simulink model "FourZones_STD2004_Buffalo_DenOcc"  (R2020a)
settings: Solver=FixedStepAuto  StartTime=20390400  StopTime=20563200  FixedStep=60  RelTol=1e-3
settings Model: Creator=zhelu  LastModifiedBy=yl3328

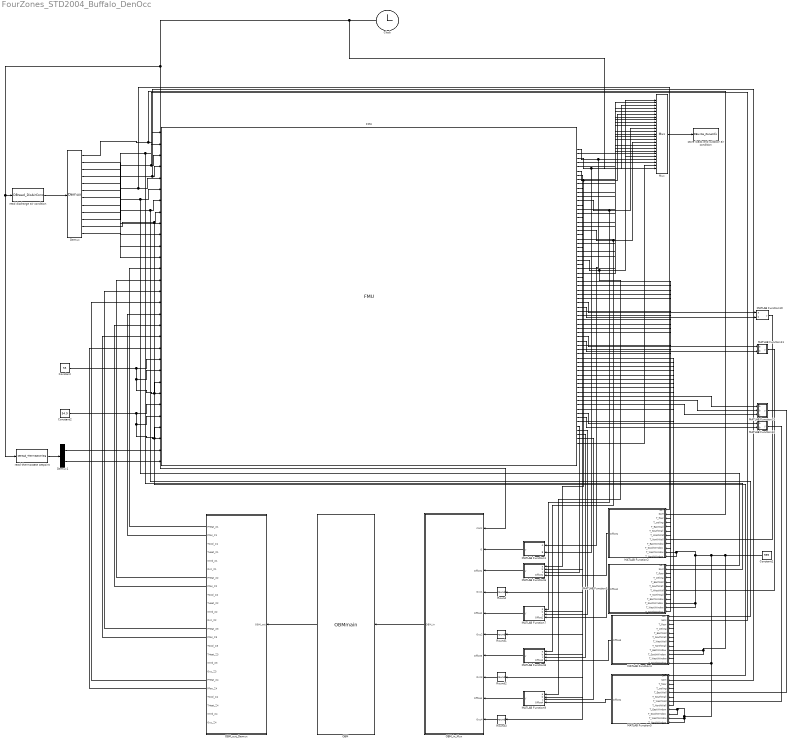
== system FourZones_STD2004_Buffalo_DenOcc ==
  Clock : Clock
  Constant : Constant  Value=55
  Constant1 : Constant  Value=999
  Constant2 : Constant  Value=54.9
  Demux : Demux  Outputs=12
  Demux1 : Demux  Outputs=2
  FMU : FMU  FMUName=ASHRAE901_OfficeMedium_STD2004_BuffaloBaseline_ARP_Cooling_dense.fmu  FMUMode=CoSimulation
      mask Type: ASHRAE901_OfficeMedium_STD2004_BuffaloBaseline.ARP_Cooling.idf [Co-Simulation, v2.0]
      mask Display:
      | disp('ASHRAE901_OfficeMedium_STD2004_BuffaloBaseline.ARP_Cooling.idf');
      | port_label('output',1,'T_out');
      | port_label('output',2,'DewpointT_out');
      | port_label('output',3,'RH_out');
      | port_label('output',4,'ConfRoom_Mid_2 ZN_SenLoads');
      | port_label('output',5,'ConfRoom_Mid_2 ZN_LatLoads');
      | port_label('output',6,'ConfRoom_Mid_2 ZN_Temp');
      | port_label('output',7,'ConfRoom_Mid_2 ZN_RadTemp');
      | port_label('output',8,'ConfRoom_Mid_2 ZN_DewpointT');
      | port_label('output',9,'ConfRoom_Mid_2 ZN_HumdRat');
      | port_label('output',10,'ConfRoom_Mid_2 ZN_Occ');
      | port_label('output',11,'EnclosedOffice_Mid_2 ZN_SenLoads');
      | port_label('output',12,'EnclosedOffice_Mid_2 ZN_LatLoads');
      | port_label('output',13,'EnclosedOffice_Mid_2 ZN_Temp');
      | port_label('output',14,'EnclosedOffice_Mid_2 ZN_RadTemp');
      | port_label('output',15,'EnclosedOffice_Mid_2 ZN_DewpointT');
      | port_label('output',16,'EnclosedOffice_Mid_2 ZN_HumdRat');
      | port_label('output',17,'EnclosedOffice_Mid_2 ZN_Occ');
      | port_label('output',18,'EnclosedOffice_Mid_5 ZN_SenLoads');
      | port_label('output',19,'EnclosedOffice_Mid_5 ZN_LatLoads');
      | port_label('output',20,'EnclosedOffice_Mid_5 ZN_Temp');
      | port_label('output',21,'EnclosedOffice_Mid_5 ZN_RadTemp');
      | port_label('output',22,'EnclosedOffice_Mid_5 ZN _DewpointT');
      | port_label('output',23,'EnclosedOffice_Mid_5 ZN_HumdRat');
      | port_label('output',24,'EnclosedOffice_Mid_5 ZN_Occ');
      | port_label('output',25,'OpenOffice_Mid_1 ZN_SenLoads');
      | port_label('output',26,'OpenOffice_Mid_1 ZN_LatLoads');
      | port_label('output',27,'OpenOffice_Mid_1 ZN_Temp');
      | port_label('output',28,'OpenOffice_Mid_1 ZN_RadTemp');
      | port_label('output',29,'OpenOffice_Mid_1 ZN_DewpointT');
      | port_label('output',30,'OpenOffice_Mid_1 ZN_HumdRat');
      | port_label('output',31,'OpenOffice_Mid_1 ZN_Occ');
      | port_label('output',32,'CONFROOM_MID_2_ZN_FLOOR_T');
      | port_label('output',33,'CONFROOM_MID_2_ZN_CEILING_T');
      | port_label('output',34,'CONFROOM_MID_2_ZN_WALL_EAST_T');
      | port_label('output',35,'CONFROOM_MID_2_ZN_WALL_SOUTH_T');
      | port_label('output',36,'CONFROOM_MID_2_ZN_WALL_WEST_T');
      | port_label('output',37,'CONFROOM_MID_2_ZN_WALL_NORTH_1_T');
      | port_label('output',38,'CONFROOM_MID_2_ZN_WALL_NORTH_2_T');
      | port_label('output',39,'CONFROOM_MID_2_ZN_WALL_EAST_WINDOW_T');
      | port_label('output',40,'CONFROOM_MID_2_ZN_WALL_SOUTH_WINDOW_T');
      | port_label('output',41,'ENCLOSEDOFFICE_MID_2_ZN_FLOOR_T');
      | port_label('output',42,'ENCLOSEDOFFICE_MID_2_ZN_CEILING_T');
      | port_label('output',43,'ENCLOSEDOFFICE_MID_2_ZN_WALL_EAST_T');
      | port_label('output',44,'ENCLOSEDOFFICE_MID_2_ZN_WALL_SOUTH_T');
      | port_label('output',45,'ENCLOSEDOFFICE_MID_2_ZN_WALL_WEST_1_T');
      | port_label('output',46,'ENCLOSEDOFFICE_MID_2_ZN_WALL_WEST_2_T');
      | port_label('output',47,'ENCLOSEDOFFICE_MID_2_ZN_WALL_NORTH_T');
      | port_label('output',48,'ENCLOSEDOFFICE_MID_2_ZN_WALL_NORTH_WINDOW_T');
      | port_label('output',49,'ENCLOSEDOFFICE_MID_2_ZN_WALL_EAST_WINDOW_T');
      | port_label('output',50,'ENCLOSEDOFFICE_MID_5_ZN_FLOOR_T');
      | port_label('output',51,'ENCLOSEDOFFICE_MID_5_ZN_CEILING_T');
      | port_label('output',52,'ENCLOSEDOFFICE_MID_5_ZN_WALL_EAST_T');
      | port_label('output',53,'ENCLOSEDOFFICE_MID_5_ZN_WALL_SOUTH_T');
      | port_label('output',54,'ENCLOSEDOFFICE_MID_5_ZN_WALL_WEST_T');
      | port_label('output',55,'ENCLOSEDOFFICE_MID_5_ZN_WALL_NORTH_T');
      | port_label('output',56,'ENCLOSEDOFFICE_MID_5_ZN_WALL_WEST_WINDOW_T');
      | port_label('output',57,'OPENOFFICE_MID_1_ZN_FLOOR_T');
      | port_label('output',58,'OPENOFFICE_MID_1_ZN_CEILING_T');
      | port_label('output',59,'OPENOFFICE_MID_1_ZN_WALL_EAST_1_T');
      | port_label('output',60,'OPENOFFICE_MID_1_ZN_WALL_EAST_2_T');
      | port_label('output',61,'OPENOFFICE_MID_1_ZN_WALL_EAST_3_T');
      | port_label('output',62,'OPENOFFICE_MID_1_ZN_WALL_SOUTH_T');
      | port_label('output',63,'OPENOFFICE_MID_1_ZN_WALL_WEST_1_T');
      | port_label('output',64,'OPENOFFICE_MID_1_ZN_WALL_WEST_2_T');
      | port_label('output',65,'OPENOFFICE_MID_1_ZN_WALL_NORTH_T');
      | port_label('output',66,'ConfRoom_Mid_2 ZN_RelaHumd');
      | port_label('output',67,'EnclosedOffice_Mid_2 ZN_RelaHumd');
      | port_label('output',68,'EnclosedOffice_Mid_5 ZN_RelaHumd');
      | port_label('output',69,'OpenOffice_Mid_1 ZN_RelaHumd');
      | port_label('output',70,'w_out');
      | port_label('input',1,'ConfRoom_Mid_2 ZN SupplyFlow');
      | port_label('input',2,'EnclosedOffice_Mid_2 ZN SupplyFlow');
      | port_label('input',3,'EnclosedOffice_Mid_5 ZN SupplyFlow');
      | port_label('input',4,'OpenOffice_Mid_1 ZN SupplyFlow');
      | port_label('input',5,'ConfRoom_Mid_2 ZN SupplyTemp');
      | port_label('input',6,'EnclosedOffice_Mid_2 ZN SupplyTemp');
      | port_label('input',7,'EnclosedOffice_Mid_5 ZN SupplyTemp');
      | port_label('input',8,'OpenOffice_Mid_1 ZN SupplyTemp');
      | port_label('input',9,'ConfRoom_Mid_2 ZN SupplyHumd');
      | port_label('input',10,'EnclosedOffice_Mid_2 ZN SupplyHumd');
      | port_label('input',11,'EnclosedOffice_Mid_5 ZN SupplyHumd');
      | port_label('input',12,'OpenOffice_Mid_1 ZN SupplyHumd');
      | port_label('input',13,'ConfRoom_Mid_2 ZN_PHeat');
      | port_label('input',14,'EnclosedOffice_Mid_2 ZN_PHeat');
      | port_label('input',15,'EnclosedOffice_Mid_5 ZN_PHeat');
      | port_label('input',16,'OpenOffice_Mid_1 ZN_PHeat');
      | port_label('input',17,'ConfRoom_Mid_2 ZN_PFan');
      | port_label('input',18,'EnclosedOffice_Mid_2 ZN_PFan');
      | port_label('input',19,'EnclosedOffice_Mid_5 ZN_PFan');
      | port_label('input',20,'OpenOffice_Mid_1 ZN_PFan');
      | port_label('input',21,'ConfRoom_Mid_2 ZN_TCool');
      | port_label('input',22,'EnclosedOffice_Mid_2 ZN_TCool');
      | port_label('input',23,'EnclosedOffice_Mid_5 ZN_TCool');
      | port_label('input',24,'OpenOffice_Mid_1 ZN_TCool');
      | port_label('input',25,'ConfRoom_Mid_2 ZN_THeat');
      | port_label('input',26,'EnclosedOffice_Mid_2 ZN_THeat');
      | port_label('input',27,'EnclosedOffice_Mid_5 ZN_THeat');
      | port_label('input',28,'OpenOffice_Mid_1 ZN_THeat');
      | port_label('input',29,'OtherZN_TC');
      | port_label('input',30,'OtherZN_TH');
  MATLAB Function1 : MATLAB Function  TreatAsAtomicUnit=on
  MATLAB Function10 : MATLAB Function  TreatAsAtomicUnit=on
  MATLAB Function11 : MATLAB Function  TreatAsAtomicUnit=on
  MATLAB Function12 : MATLAB Function  TreatAsAtomicUnit=on
  MATLAB Function13 : MATLAB Function  TreatAsAtomicUnit=on
  MATLAB Function2 : MATLAB Function  TreatAsAtomicUnit=on
  MATLAB Function3 : MATLAB Function  TreatAsAtomicUnit=on
  MATLAB Function4 : MATLAB Function  TreatAsAtomicUnit=on
  MATLAB Function5 : MATLAB Function  TreatAsAtomicUnit=on
  MATLAB Function6 : MATLAB Function  TreatAsAtomicUnit=on
  MATLAB Function7 : MATLAB Function  TreatAsAtomicUnit=on
  MATLAB Function8 : MATLAB Function  TreatAsAtomicUnit=on
  MATLAB Function9 : MATLAB Function  TreatAsAtomicUnit=on
  Mux : Mux  Inputs=25
  OBM : M-S-Function  FunctionName=OBMmain
  OBM_in_Mux : MATLAB Function  TreatAsAtomicUnit=on
  OBM_out_Demux : MATLAB Function  TreatAsAtomicUnit=on
  Round{,1..3} (4 alike) : Rounding  Operator=round
  read discharge air condition : M-S-Function  FunctionName=DBread_DisAirCond
  read thermostate setpoint : M-S-Function  FunctionName=DBread_ThermSptCtrlSig
  store loads and outdoor air condition : M-S-Function  FunctionName=DBwrite_ZoneInfo
  wires:
  Constant1/1 -> MATLAB Function5/11(T_WestWindow), MATLAB Function5/12(T_NorthWindow), MATLAB Function5/9(T_EastWindow), MATLAB Function5/10(T_SouthWindow), MATLAB Function4/12(T_NorthWindow), MATLAB Function3/10(T_SouthWindow), MATLAB Function3/11(T_WestWindow), MATLAB Function2/12(T_NorthWindow), MATLAB Function2/11(T_WestWindow), MATLAB Function4/10(T_SouthWindow), MATLAB Function4/9(T_EastWindow)
  FMU/1 -> MATLAB Function1/1(A), Mux/1
  MATLAB Function10/1(y) -> MATLAB Function2/8(T_NorthWall)
  MATLAB Function11/1(y) -> MATLAB Function3/7(T_WestWall)
  MATLAB Function12/1(y) -> MATLAB Function5/7(T_WestWall)
  MATLAB Function13/1(y) -> MATLAB Function5/5(T_EastWall)
  Constant/1 -> FMU/24, FMU/23, FMU/22, FMU/21
  Constant2/1 -> FMU/28, FMU/27, FMU/26, FMU/25
  Mux/1 -> store loads and outdoor air condition/1
  read discharge air condition/1 -> Demux/1
  Demux/1 -> MATLAB Function2/2(SAM), FMU/1
  Demux/4 -> MATLAB Function3/2(SAM), FMU/2
  Demux/7 -> MATLAB Function4/2(SAM), FMU/3
  Demux/10 -> MATLAB Function5/2(SAM), FMU/4
  Demux/2 -> MATLAB Function2/1(SAT), FMU/5
  Demux/5 -> MATLAB Function3/1(SAT), FMU/6
  Demux/8 -> MATLAB Function4/1(SAT), FMU/7
  Demux/11 -> MATLAB Function5/1(SAT), FMU/8
  Demux/3 -> FMU/9
  Demux/6 -> FMU/10
  Demux/9 -> FMU/11
  Demux/12 -> FMU/12
  Clock/1 -> Mux/25, read thermostate setpoint/1, read discharge air condition/1, OBM_in_Mux/1(clock)
  MATLAB Function1/1(y) -> OBM_in_Mux/2(O)
  MATLAB Function6/1(y) -> OBM_in_Mux/3(Office1)
  Round/1 -> OBM_in_Mux/4(Occ1)
  MATLAB Function7/1(y) -> OBM_in_Mux/5(Office2)
  Round1/1 -> OBM_in_Mux/6(Occ2)
  MATLAB Function8/1(y) -> OBM_in_Mux/7(Office3)
  Round2/1 -> OBM_in_Mux/8(Occ3)
  MATLAB Function9/1(y) -> OBM_in_Mux/9(Office4)
  Round3/1 -> OBM_in_Mux/10(Occ4)
  OBM_out_Demux/1(PHeat_Z1) -> FMU/13
  OBM_out_Demux/2(PFan_Z1) -> FMU/17
  OBM_out_Demux/7(PHeat_Z2) -> FMU/14
  OBM_out_Demux/8(PFan_Z2) -> FMU/18
  OBM_out_Demux/13(PHeat_Z3) -> FMU/15
  OBM_out_Demux/14(PFan_Z3) -> FMU/19
  OBM_out_Demux/19(PHeat_Z4) -> FMU/16
  OBM_out_Demux/20(PFan_Z4) -> FMU/20
  OBM_in_Mux/1(OBM_in) -> OBM/1
  OBM/1 -> OBM_out_Demux/1(OBM_out)
  FMU/37 -> MATLAB Function10/1(a)
  FMU/38 -> MATLAB Function10/2(b)
  FMU/32 -> MATLAB Function2/3(T_floor)
  FMU/33 -> MATLAB Function2/4(T_ceiling)
  FMU/34 -> MATLAB Function2/5(T_EastWall)
  FMU/35 -> MATLAB Function2/6(T_SouthWall)
  FMU/36 -> MATLAB Function2/7(T_WestWall)
  FMU/39 -> MATLAB Function2/9(T_EastWindow)
  FMU/40 -> MATLAB Function2/10(T_SouthWindow)
  FMU/41 -> MATLAB Function3/3(T_floor)
  FMU/42 -> MATLAB Function3/4(T_ceiling)
  FMU/43 -> MATLAB Function3/5(T_EastWall)
  FMU/44 -> MATLAB Function3/6(T_SouthWall)
  FMU/45 -> MATLAB Function11/1(a)
  FMU/46 -> MATLAB Function11/2(b)
  FMU/47 -> MATLAB Function3/8(T_NorthWall)
  FMU/49 -> MATLAB Function3/9(T_EastWindow)
  FMU/48 -> MATLAB Function3/12(T_NorthWindow)
  FMU/50 -> MATLAB Function4/3(T_floor)
  FMU/51 -> MATLAB Function4/4(T_ceiling)
  FMU/52 -> MATLAB Function4/5(T_EastWall)
  FMU/53 -> MATLAB Function4/6(T_SouthWall)
  FMU/54 -> MATLAB Function4/7(T_WestWall)
  FMU/55 -> MATLAB Function4/8(T_NorthWall)
  FMU/56 -> MATLAB Function4/11(T_WestWindow)
  FMU/57 -> MATLAB Function5/3(T_floor)
  FMU/58 -> MATLAB Function5/4(T_ceiling)
  FMU/59 -> MATLAB Function13/1(a)
  FMU/60 -> MATLAB Function13/2(b)
  FMU/61 -> MATLAB Function13/3(c)
  FMU/62 -> MATLAB Function5/6(T_SouthWall)
  FMU/65 -> MATLAB Function5/8(T_NorthWall)
  FMU/63 -> MATLAB Function12/1(a)
  FMU/64 -> MATLAB Function12/2(b)
  FMU/10 -> Round/1
  FMU/17 -> Round1/1
  FMU/24 -> Round2/1
  FMU/31 -> Round3/1
  FMU/3 -> Mux/3, MATLAB Function1/2(B)
  FMU/5 -> Mux/5
  FMU/6 -> Mux/6, MATLAB Function6/1(a)
  FMU/7 -> MATLAB Function6/2(b)
  FMU/9 -> Mux/8
  FMU/13 -> Mux/11, MATLAB Function7/1(a)
  FMU/14 -> MATLAB Function7/2(b)
  FMU/16 -> Mux/13
  FMU/20 -> Mux/16, MATLAB Function8/1(a)
  FMU/21 -> MATLAB Function8/2(b)
  FMU/23 -> Mux/18
  FMU/27 -> Mux/21, MATLAB Function9/1(a)
  FMU/28 -> MATLAB Function9/2(b)
  FMU/30 -> Mux/23
  FMU/2 -> Mux/2
  FMU/4 -> Mux/4
  FMU/8 -> Mux/7
  FMU/11 -> Mux/9
  FMU/12 -> Mux/10
  FMU/15 -> Mux/12
  FMU/18 -> Mux/14
  FMU/19 -> Mux/15
  FMU/22 -> Mux/17
  FMU/25 -> Mux/19
  FMU/26 -> Mux/20
  FMU/29 -> Mux/22
  MATLAB Function2/1(Office1) -> MATLAB Function6/4(Office1)
  MATLAB Function3/1(Office2) -> MATLAB Function7/4(Office2)
  MATLAB Function4/1(Office3) -> MATLAB Function8/4(Office3)
  MATLAB Function5/1(Office4) -> MATLAB Function9/4(Office4)
  FMU/66 -> MATLAB Function6/3(c)
  FMU/67 -> MATLAB Function7/3(c)
  FMU/68 -> MATLAB Function8/3(c)
  FMU/69 -> MATLAB Function9/3(c)
  FMU/70 -> Mux/24
  read thermostate setpoint/1 -> Demux1/1
  Demux1/1 -> FMU/29
  Demux1/2 -> FMU/30

== matlab function FourZones_STD2004_Buffalo_DenOcc/MATLAB Function5 ==
  data: SAT input; SAM input; T_floor input; Office4 output; T_ceiling input; T_EastWall input; T_SouthWall input; T_WestWall input; T_NorthWall input; T_EastWindow input; T_SouthWindow input; T_WestWindow input; T_NorthWindow input
function Office4 = fcn(SAT,SAM,T_floor,T_ceiling,T_EastWall,T_SouthWall,T_WestWall,T_NorthWall,...
    T_EastWindow,T_SouthWindow,T_WestWindow,T_NorthWindow)
Office4=[SAT,SAM,T_floor,T_ceiling,T_EastWall,T_SouthWall,T_WestWall,T_NorthWall,...
    T_EastWindow,T_SouthWindow,T_WestWindow,T_NorthWindow];

== matlab function FourZones_STD2004_Buffalo_DenOcc/MATLAB Function6 ==
  data: a input; y output; b input; c input; Office1 input
function y = fcn(a, b, c, Office1)

y = [a b c Office1];

== matlab function FourZones_STD2004_Buffalo_DenOcc/MATLAB Function7 ==
  data: a input; y output; b input; c input; Office2 input
function y = fcn(a, b, c, Office2)

y = [a b c Office2];

== matlab function FourZones_STD2004_Buffalo_DenOcc/MATLAB Function8 ==
  data: a input; y output; b input; c input; Office3 input
function y = fcn(a, b, c, Office3)

y = [a b c Office3];

== matlab function FourZones_STD2004_Buffalo_DenOcc/MATLAB Function9 ==
  data: a input; y output; b input; c input; Office4 input
function y = fcn(a, b, c, Office4)

y = [a b c Office4];

== matlab function FourZones_STD2004_Buffalo_DenOcc/MATLAB Function10 ==
  data: a input; y output; b input
function y = fcn(a,b)
u=(a+b)/2;
y = u;

== matlab function FourZones_STD2004_Buffalo_DenOcc/MATLAB Function11 ==
  data: a input; y output; b input
function y = fcn(a,b)
u=(a+b)/2;
y = u;

== matlab function FourZones_STD2004_Buffalo_DenOcc/MATLAB Function12 ==
  data: a input; y output; b input
function y = fcn(a,b)
u=(a+b)/2;
y = u;

== matlab function FourZones_STD2004_Buffalo_DenOcc/MATLAB Function13 ==
  data: a input; y output; b input; c input
function y = fcn(a,b,c)
u=(a+b+c)/3;
y = u;

== matlab function FourZones_STD2004_Buffalo_DenOcc/OBM_out_Demux ==
  data: OBM_out input; PHeat_Z1 output; PFan_Z1 output; TCool_Z1 output; THeat_Z1 output; Wind_Z1 output; Occ_Z1 output; PHeat_Z2 output; PFan_Z2 output; TCool_Z2 output; THeat_Z2 output; Wind_Z2 output; Occ_Z2 output; PHeat_Z3 output; PFan_Z3 output; TCool_Z3 output; THeat_Z3 output; Wind_Z3 output; Occ_Z3 output; PHeat_Z4 output; PFan_Z4 output; TCool_Z4 output; THeat_Z4 output; Wind_Z4 output; Occ_Z4 output
function [PHeat_Z1,PFan_Z1,TCool_Z1,THeat_Z1,Wind_Z1,Occ_Z1,...
    PHeat_Z2,PFan_Z2,TCool_Z2,THeat_Z2,Wind_Z2,Occ_Z2,...
    PHeat_Z3,PFan_Z3,TCool_Z3,THeat_Z3,Wind_Z3,Occ_Z3,...
    PHeat_Z4,PFan_Z4,TCool_Z4,THeat_Z4,Wind_Z4,Occ_Z4] = fcn(OBM_out)

PHeat_Z1 = OBM_out(1);
PFan_Z1 = OBM_out(2);
TCool_Z1 = OBM_out(3);
THeat_Z1 = OBM_out(4);
Wind_Z1 = OBM_out(5);
Occ_Z1 = OBM_out(6);
PHeat_Z2 = OBM_out(7);
PFan_Z2 = OBM_out(8);
TCool_Z2 = OBM_out(9);
THeat_Z2 = OBM_out(10);
Wind_Z2 = OBM_out(11);
Occ_Z2 = OBM_out(12);
PHeat_Z3 = OBM_out(13);
PFan_Z3 = OBM_out(14);
TCool_Z3 = OBM_out(15);
THeat_Z3 = OBM_out(16);
Wind_Z3 = OBM_out(17);
Occ_Z3 = OBM_out(18);
PHeat_Z4 = OBM_out(19);
PFan_Z4 = OBM_out(20);
TCool_Z4 = OBM_out(21);
THeat_Z4 = OBM_out(22);
Wind_Z4 = OBM_out(23);
Occ_Z4 = OBM_out(24);

== matlab function FourZones_STD2004_Buffalo_DenOcc/MATLAB Function1 ==
  data: A input; y output; B input
function y = fcn(A,B)

y = [A B];

== matlab function FourZones_STD2004_Buffalo_DenOcc/OBM_in_Mux ==
  data: clock input; OBM_in output; O input; Office1 input; Occ1 input; Office2 input; Occ2 input; Office3 input; Occ3 input; Office4 input; Occ4 input
function OBM_in = fcn(clock,O,Office1,Occ1,Office2,Occ2,...
    Office3,Occ3,Office4,Occ4)
% Assemble OBM inputs
OBM_in=[clock,O,Office1,Occ1,Office2,Occ2,Office3,Occ3,Office4,Occ4]';

== matlab function FourZones_STD2004_Buffalo_DenOcc/MATLAB Function2 ==
  data: SAT input; SAM input; T_floor input; Office1 output; T_ceiling input; T_EastWall input; T_SouthWall input; T_WestWall input; T_NorthWall input; T_EastWindow input; T_SouthWindow input; T_WestWindow input; T_NorthWindow input
function Office1 = fcn(SAT,SAM,T_floor,T_ceiling,T_EastWall,T_SouthWall,T_WestWall,T_NorthWall,...
    T_EastWindow,T_SouthWindow,T_WestWindow,T_NorthWindow)
Office1=[SAT,SAM,T_floor,T_ceiling,T_EastWall,T_SouthWall,T_WestWall,T_NorthWall,...
    T_EastWindow,T_SouthWindow,T_WestWindow,T_NorthWindow];

== matlab function FourZones_STD2004_Buffalo_DenOcc/MATLAB Function3 ==
  data: SAT input; SAM input; T_floor input; Office2 output; T_ceiling input; T_EastWall input; T_SouthWall input; T_WestWall input; T_NorthWall input; T_EastWindow input; T_SouthWindow input; T_WestWindow input; T_NorthWindow input
function Office2 = fcn(SAT,SAM,T_floor,T_ceiling,T_EastWall,T_SouthWall,T_WestWall,T_NorthWall,...
    T_EastWindow,T_SouthWindow,T_WestWindow,T_NorthWindow)
Office2=[SAT,SAM,T_floor,T_ceiling,T_EastWall,T_SouthWall,T_WestWall,T_NorthWall,...
    T_EastWindow,T_SouthWindow,T_WestWindow,T_NorthWindow];

== matlab function FourZones_STD2004_Buffalo_DenOcc/MATLAB Function4 ==
  data: SAT input; SAM input; T_floor input; Office3 output; T_ceiling input; T_EastWall input; T_SouthWall input; T_WestWall input; T_NorthWall input; T_EastWindow input; T_SouthWindow input; T_WestWindow input; T_NorthWindow input
function Office3 = fcn(SAT,SAM,T_floor,T_ceiling,T_EastWall,T_SouthWall,T_WestWall,T_NorthWall,...
    T_EastWindow,T_SouthWindow,T_WestWindow,T_NorthWindow)
Office3=[SAT,SAM,T_floor,T_ceiling,T_EastWall,T_SouthWall,T_WestWall,T_NorthWall,...
    T_EastWindow,T_SouthWindow,T_WestWindow,T_NorthWindow];
